simulink model "hornet_sim_1D"  (R2026a)
settings: Solver=VariableStepAuto
values from neighbouring files (symbols this model uses):
  g = 9.81    [Hornet_6DOF_FS_init.m]    (also in hornet_sim_1D_init.m)
  Kd = 10    [Hornet_6DOF_FS_init.m]    (also in hornet_sim_1D_init.m)
  Kp = 10    [Hornet_6DOF_FS_init.m]    (also in hornet_sim_1D_init.m)
  m = 100    [Hornet_6DOF_FS_init.m]    (also in hornet_sim_1D_init.m = 2)
  m_true = m    (= 2)    [hornet_sim_1D_init.m]
  tau = 0.2    [Hornet_6DOF_FS_init.m]    (also in hornet_sim_1D_init.m)
  Tmax = 400    [Hornet_6DOF_FS_init.m]    (also in hornet_sim_1D_init.m = 32)
  Tmin = 0    [Hornet_6DOF_FS_init.m]    (also in hornet_sim_1D_init.m)
  vx0 = 0    [Hornet_6DOF_FS_init.m]    (also in hornet_sim_1D_init.m)
  x0 = 0    [Hornet_6DOF_FS_init.m]    (also in hornet_sim_1D_init.m = 1)
settings Model: Creator=11and  LastModifiedBy=11and

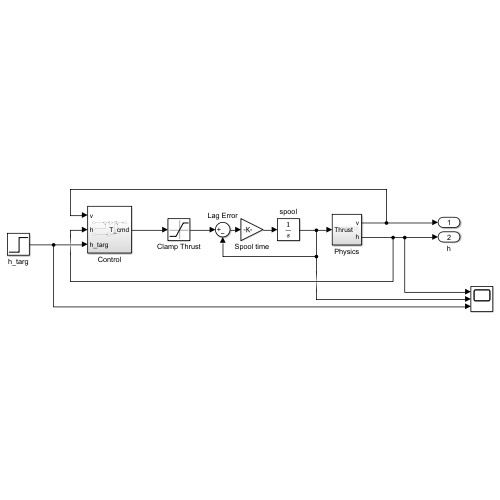
[thumbnail: Simulink's stored preview of the top-level diagram]
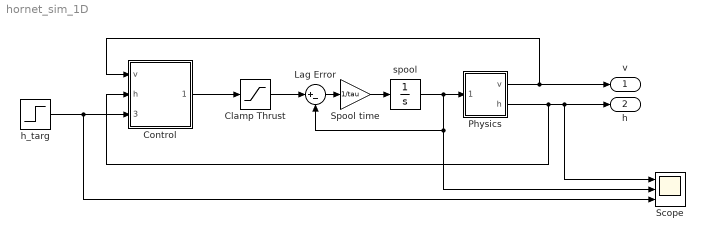
== system hornet_sim_1D ==
  Clamp Thrust : Saturate  UpperLimit=Tmax  LowerLimit=Tmin
  Control : Subsystem
  Lag Error : Sum  Inputs=|+-
  Physics : Subsystem
  Scope : Scope  NumInputPorts=3
      settings: ActiveDisplayYMinimum=-16.062341743089117  ActiveDisplayYMaximum=31.824437612543942
  Spool time : Gain  Gain=1/tau
  h_targ : Step  Time=15  InitialValue=x_targ  FinalValue=x_targ  SampleTime=0
  spool : Integrator
  v : Outport
  h : Outport  Port=2
  wires:
  Physics/2(h) -> Control/2(h), Scope/1, h/1
  Physics/1(v) -> Control/1(v), v/1
  spool/1 -> Scope/2, Lag Error/2, Physics/1(Thrust)
  Clamp Thrust/1 -> Lag Error/1
  Spool time/1 -> spool/1
  Lag Error/1 -> Spool time/1
  h_targ/1 -> Scope/3, Control/3(h_targ)
  Control/1(T_cmd) -> Clamp Thrust/1

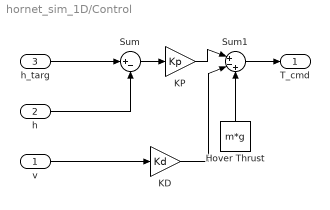
== system hornet_sim_1D/Control ==
  v : Inport
  h : Inport  Port=2
  h_targ : Inport  Port=3
  Hover Thrust : Constant  Value=m*g
  KD : Gain  Gain=Kd
  KP : Gain  Gain=Kp
  Sum : Sum  Inputs=|+-
  Sum1 : Sum  Inputs=|+-+
  T_cmd : Outport
  wires:
  KP/1 -> Sum1/1
  Sum/1 -> KP/1
  h_targ/1 -> Sum/1
  KD/1 -> Sum1/2
  h/1 -> Sum/2
  v/1 -> KD/1
  Hover Thrust/1 -> Sum1/3
  Sum1/1 -> T_cmd/1

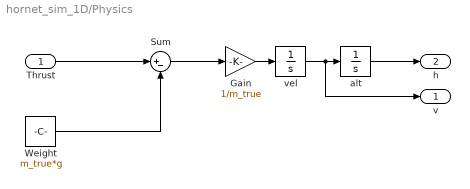
== system hornet_sim_1D/Physics ==
  Thrust : Inport
  Gain : Gain  Gain=1/m_true
  Sum : Sum  Inputs=|+-
  Weight : Constant  Value=m_true*g
  alt : Integrator  InitialCondition=x0
  vel : Integrator  InitialCondition=vx0
  v : Outport
  h : Outport  Port=2
  wires:
  Weight/1 -> Sum/2
  vel/1 -> v/1, alt/1
  Sum/1 -> Gain/1
  alt/1 -> h/1
  Gain/1 -> vel/1
  Thrust/1 -> Sum/1
